simulink model "S_PARAM_V1"  (R2017a)
settings: Solver=VariableStepAuto  StartTime=0.0  StopTime=0.4  FixedStep=1e-6  MaxStep=1e-4  RelTol=1e-3
values from neighbouring files (symbols this model uses):
  a = 9    [M_PARAM_V1.m]    (also in M_PIL_PVSISTEM_2026_V1.m; ModTusk_V1.m)
  Alpha1 = 2*Zeta_obs*wn_obs    (= 2)    [M_PARAM_V1.m]    (also in M_PIL_PVSISTEM_2026_V1.m)
  Alpha2 = wn_obs    (= 1)    [M_PARAM_V1.m]    (also in M_PIL_PVSISTEM_2026_V1.m)
  alpha_max = 4/ts_min    (= 13333.3333333)    [M_PARAM_V1.m]    (also in M_PIL_PVSISTEM_2026_V1.m; ModTusk_V1.m)
  alpha_min = 4/ts_max    (= 259.067357513)    [M_PARAM_V1.m]    (also in M_PIL_PVSISTEM_2026_V1.m = 133.333333333; ModTusk_V1.m = 133.333333333)
  Cdc = Cdc    (= 0.0033)    [M_PARAM_V1.m]    (also in M_PIL_PVSISTEM_2026_V1.m = 0.00047)
  Cpv = Cpv    (= 0.0001)    [M_PARAM_V1.m]    (also in M_PIL_PVSISTEM_2026_V1.m = 0.0002)
  Epsilon = Ep_cont/Ts1    [M_PARAM_V1.m]    (also in M_PIL_PVSISTEM_2026_V1.m)
  ESRCdc = ESRCdc    (= 0.2)    [M_PARAM_V1.m]    (also in M_PIL_PVSISTEM_2026_V1.m)
  ESRCpv = ESRCpv    (= 0.2)    [M_PARAM_V1.m]    (also in M_PIL_PVSISTEM_2026_V1.m)
  K1 = Kt_acker_d    [M_PARAM_V1.m]    (also in M_PIL_PVSISTEM_2026_V1.m)
  K1y2md = Kmd(1:end-1)    [M_PARAM_V1.m]    (also in M_PIL_PVSISTEM_2026_V1.m)
  Kdpwm = 1/Ucmax    (= 0.000111111111111)    [M_PARAM_V1.m]    (also in M_PIL_PVSISTEM_2026_V1.m = 1.52590218967e-05)
  KI1 = Kp1/Ti1*Ts1    (= 760)    [M_PARAM_V1.m]    (also in M_PIL_PVSISTEM_2026_V1.m = 14.4)
  Kimd = -Kmd(end)    [M_PARAM_V1.m]    (also in M_PIL_PVSISTEM_2026_V1.m)
  KP1 = Kp1-KI1/2    (= 5320)    [M_PARAM_V1.m]    (also in M_PIL_PVSISTEM_2026_V1.m = 2392.8)
  L = L    (= 0.0044)    [M_PARAM_V1.m]    (also in M_PIL_PVSISTEM_2026_V1.m = 0.1)
  RL = RL    (= 0.494)    [M_PARAM_V1.m]    (also in M_PIL_PVSISTEM_2026_V1.m = 0.3)
  Ts = Ts1    (= 0.0002)    [M_PARAM_V1.m]    (also in M_PIL_PVSISTEM_2026_V1.m)
  Ts1 = 1/Fs    (= 0.0002)    [M_PARAM_V1.m]    (also in M_PIL_PVSISTEM_2026_V1.m)
  Ucmax = 9000    [M_PARAM_V1.m]    (also in M_PIL_PVSISTEM_2026_V1.m = 65535)
  vdc = 12    [M_PARAM_V1.m]    (also in M_PIL_PVSISTEM_2026_V1.m = 1000)
undefined symbols (not defined in the file or in its folder): Acid, Lead
undefined symbols (not defined in the file): Fs
libraries: powerlib x14, electricdrivelib x1, powerlib_meascontrol x1
settings Model: ExtModeTrigDuration=10  Creator=dricl  LastModifiedBy=dricl
settings OptimizationCC: PassReuseOutputArgsAs=Individual arguments  MaxStackSize=2560
settings DebuggingCC: ParameterTunabilityLossMsg=error
settings HardwareCC: ProdBitPerPointer=32  ProdBitPerSizeT=32  ProdBitPerPtrDiffT=32  ProdLargestAtomicInteger=Long  ProdLargestAtomicFloat=Double  ProdWordSize=32  ProdLongLongMode=on  ProdHWDeviceType=ARM Compatible->ARM Cortex
settings SFSimCC: MATLABDynamicMemAlloc=off
settings RTWCC: SystemTargetFile=ert.tlc  HardwareBoard=TI Concerto F28M35x (ARM Cortex-M3)  TLCOptions=-aInlineSetEventsForThisBaseRateFcn=TLC_FALSE -aSuppressMultiTaskScheduler=TLC_FALSE -aRateBasedStepFcn=1  TemplateMakefile=ert_default_tmf  Description=Embedded Coder  GenerateReport=on  Toolchain=Texas Instruments Code Composer Studio v6 (ARM)  IncludeHyperlinkInReport=on  LaunchReport=on  CreateSILPILBlock=PIL  GenerateTraceInfo=on  GenerateTraceReport=on  GenerateTraceReportSl=on  GenerateTraceReportSf=on  GenerateTraceReportEml=on
settings CodeAppCC: ForceParamTrailComments=on  IgnoreCustomStorageClasses=off  OperatorAnnotations=on  SimulinkDataObjDesc=on  SFDataObjDesc=on  MATLABFcnDesc=on  InsertBlockDesc=on  MATLABSourceComments=on

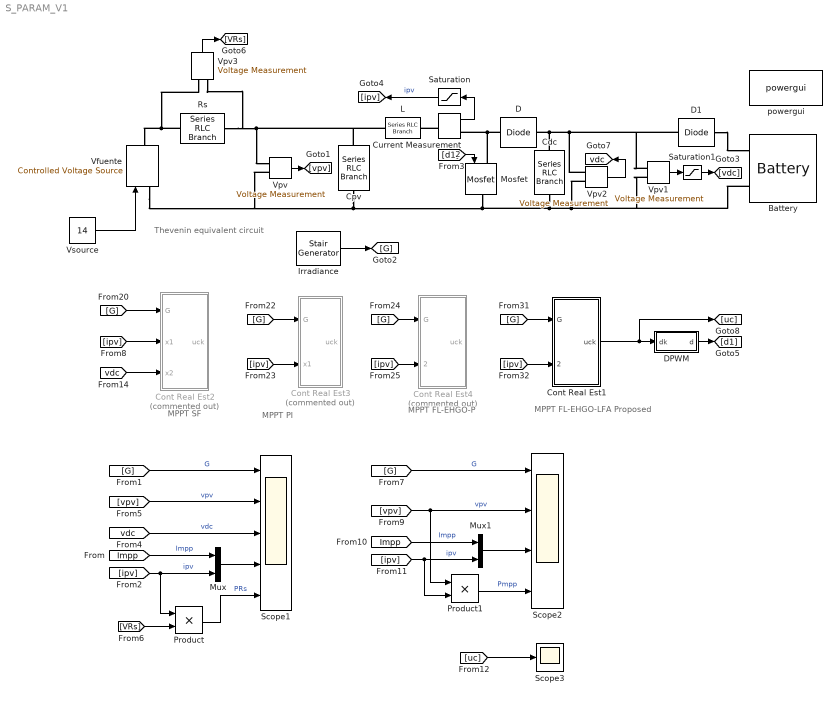
== system S_PARAM_V1 ==
  note: Thevenin equivalent circuit
  note: MPPT PI
  note: MPPT SF
  note: MPPT FL-EHGO-P
  note: MPPT FL-EHGO-LFA
      | Proposed
  Battery : electricdrivelib/Extra Sources/Battery  BatType=Lead-Acid  ShowTempParam=off  ThermalPreset=no  ShowAgeParam=off  NomV=12  NomQ=1.2  SOC=100  Batt_Tr=30  PresetModel=on  MaxQ=1.25  MinV=9  FullV=13.0658  Dis_rate=0.24  R=0.1  Normal_OP=0.37233  expZone="[12.2171        0.004]"  current=[6.5 13 32.5]  Units=Time  Tci=20  NomT=20  T2=-30  MaxQ2=4.8  FullV2=7.1  Normal_OP2=5.655  expZone2="[6.58           1]"  Rca=0.6  ti=2000  Dp=0  Neq0=0  Tsim=1e6  Ta1=25  Qeol=5.4*0.9  Reol=0.013333*1.2  Char_age=[2.3478, 3]  Dis_age=[2.3478, 10]  N1=1500  N2=10500  N3=1000  N4=1400  Ta2=45  N5=950
  Cdc : powerlib/Elements/Series RLC Branch  LConnTagsString=__new0  RConnTagsString=__new0  BranchType=RC  Resistance=ESRCdc  Inductance=1e-3  SetiL0=off  InitialCurrent=0  Capacitance=Cdc  Setx0=on  InitialVoltage=vdc_ref  Measurements=None
  Cont Real Est1 : Subsystem  Priority=7
  Cont Real Est2 : Subsystem  Priority=9  Commented=on
  Cont Real Est3 : Subsystem  Priority=7  Commented=on
  Cont Real Est4 : Subsystem  Priority=7  Commented=on
  Cpv : powerlib/Elements/Series RLC Branch  LConnTagsString=__new0  RConnTagsString=__new0  BranchType=RC  Resistance=ESRCpv  Inductance=1e-3  SetiL0=off  InitialCurrent=0  Capacitance=Cpv  Setx0=off  InitialVoltage=640.8  Measurements=None
  Current Measurement2 : powerlib/Measurements/Current Measurement  PhasorSimulation=off  OutputType=Complex  PSBequivalent=0
  D : powerlib/Power Electronics/Diode  Ron=Rondiode  Lon=0  Vf=Vfdiode  IC=0  UseSnubber=0  Rs=500  Cs=250e-9  Measurements=off
  D1 : powerlib/Power Electronics/Diode  Ron=0.001  Lon=0  Vf=0.7  IC=0  UseSnubber=0  Rs=500  Cs=250e-9  Measurements=off
  DPWM : Subsystem  AncestorBlock=plecslib_extras2/Modulators/Symmetrical PWM  mask(Symmetrical PWM){sampling=Natural (carrier starts with 0), fc=Fs, offset=0, input_limits=[0 Ucmax], output_values=[0 1]}
      mask prompts: fc "Carrier frequency (Hz):"; offset "Carrier offset (p.u.):"; input_limits "Input limits [min max]:"; output_values "Output values [off on]:"
      mask help: PWM generator with a symmetrical triangular carrier. If the input is a vector, the output is also a vector of the same width.
      mask init:
      | if numel(fc)>1 || fc<=0,
      |   error('Carrier frequency must be a positive scalar.');
      | end
      | if numel(offset)>1 || offset<0 || offset>=1,
      |   error('Carrier offset must be a scalar in the range [0; 1/fc[.');
      | end
      | if sampling == 1,
      |   offset = mod(offset+.75, 1);
      | end
      | 
      | si = [.5 mod(offset, .5)]/fc;
      mask Help: eval('plecs(''help'', ''symmetricalpwm.html'')')
      mask TypeOptions sampling: Natural (carrier starts with 0) | Natural (carrier starts with 1) | Regular (double edge) | Regular (single edge)
  Irradiance : powerlib_meascontrol/Pulse & Signal Generators/Stair Generator  t=[0, .1, .2, .3]  e=[0 1000 200 850]  Ts=0
      settings: SourceProductName=Simscape Power Systems
  L : powerlib/Elements/Series RLC Branch  LConnTagsString=__new0  RConnTagsString=__new0  BranchType=RL  Resistance=RL  Inductance=L  SetiL0=off  InitialCurrent=0  Capacitance=1e-6  Setx0=off  InitialVoltage=0  Measurements=None
  Mosfet : powerlib/Power Electronics/Mosfet  Ron=Ronfet  Lon=0  Rd=0  Vfd=0  IC=0  Rs=1e5  Cs=inf  Measurements=off
  Mux : Mux  Inputs=2
  Mux1 : Mux  Inputs=2
  Product : Product
  Product1 : Product
  Rs : powerlib/Elements/Series RLC Branch  LConnTagsString=__new0  RConnTagsString=__new0  BranchType=R  Resistance=2  Inductance=1e-3  SetiL0=off  InitialCurrent=0  Capacitance=Cpv  Setx0=off  InitialVoltage=640.8  Measurements=None
  Saturation : Saturate  UpperLimit=inf  LowerLimit=0
  Saturation1 : Saturate  UpperLimit=20  LowerLimit=0
  Scope1 : Scope  NumInputPorts=5
  Scope2 : Scope  NumInputPorts=4
  Scope3 : Scope
  Vfuente : powerlib/Electrical Sources/Controlled Voltage Source  Initialize=on  Source_Type=AC  Amplitude=0  Phase=0  Frequency=0  Measurements=None
  Vpv{,1..3} (4 alike) : powerlib/Measurements/Voltage Measurement  PhasorSimulation=off  OutputType=Complex  PSBequivalent=0
  Vsource : Constant  Value=14
  powergui : powerlib/powergui  Priority=1  SimulationMode=Continuous  SampleTime=50e-6  frequency=60  Iterations=50  frequencyindice=0  Pbase=100e6  ErrMax=1e-4  UnitsV=kV  UnitsW=MW  buscounter=0  FunctionMessages=off  echomessages=off  EnableUseOfTLC=off  CurrentSourceSwitches=off  DisableSnubberDevices=off  DisableRonSwitches=off  DisableVfSwitches=off  DisplayEquations=off  SolverType=Tustin/Backward Euler (TBE)  Interpol=off  ExternalGateDelay=off  methode=off  Ts=100  x0status=blocks  SPID=on  SwTol=0  HookPort=off  RestoreLinks=warning  ResistiveCurrentMeasurement=off  Frange=[0:2:500]  Ylog=off  Xlog=on  ShowGrid=off  save=off  variable=ZData  structure=0  ZoomFFT=off  StartTime=0.0  cycles=1  DisplayStyle=1  fundamental=60  FreqAxis=off  MaxFrequency=1000  frequencyindicesteady=1  RmsSteady=1  display=off
  tag scope: vdc=global
  wires:
  Vpv2/1 -> [vdc]
  DPWM/1(d) -> [d1]
  Saturation/1 -> [ipv]  "ipv"
  Vpv/1 -> [vpv]
  [d1] -> Mosfet/1
  Current Measurement2/1 -> Saturation/1
  [ipv] -> Product/1, Mux/2  "ipv"
  [Impp] -> Mux/1  "Impp"
  [G] -> Scope1/1  "G"
  Vpv1/1 -> Saturation1/1
  Saturation1/1 -> [vdc]
  [vdc] -> Scope1/3  "vdc"
  Mux/1 -> Scope1/4
  [vpv] -> Scope1/2  "vpv"
  Vpv3/1 -> [VRs]
  Product/1 -> Scope1/5  "PRs"
  [VRs] -> Product/2
  [Impp] -> Mux1/1  "Impp"
  [ipv] -> Product1/2, Mux1/2  "ipv"
  [G] -> Scope2/1  "G"
  [vpv] -> Product1/1, Scope2/2  "vpv"
  Mux1/1 -> Scope2/3
  Product1/1 -> Scope2/4  "Pmpp"
  Vsource/1 -> Vfuente/1
  Irradiance/1 -> [G]
  [G] -> Cont Real Est2/1(G)
  [ipv] -> Cont Real Est2/2(x1)
  [vdc] -> Cont Real Est2/3(x2)
  [ipv] -> Cont Real Est1/2(x1 = ipv)
  [G] -> Cont Real Est1/1(G)
  [uc] -> Scope3/1
  [G] -> Cont Real Est4/1(G)
  [ipv] -> Cont Real Est4/2(x1 = ipv)
  [G] -> Cont Real Est3/1(G)
  [ipv] -> Cont Real Est3/2(x1)
  Cont Real Est1/1(uck) -> [uc], DPWM/1(dk)
  connections:
  Cpv/LConn1 -- L/LConn1 -- Vpv3/LConn2 -- Rs/RConn1 -- Vpv/LConn1
  Cdc/RConn1 -- Vpv1/LConn2 -- Battery/LConn2 -- Vpv2/LConn2 -- Vfuente/LConn1 -- Vpv/LConn2 -- Cpv/RConn1 -- Mosfet/RConn1
  D/RConn1 -- Cdc/LConn1 -- Vpv1/LConn1 -- D1/LConn1 -- Vpv2/LConn1
  D/LConn1 -- Mosfet/LConn1 -- Current Measurement2/RConn1
  Current Measurement2/LConn1 -- L/RConn1
  D1/RConn1 -- Battery/LConn1
  Rs/LConn1 -- Vpv3/LConn1 -- Vfuente/RConn1

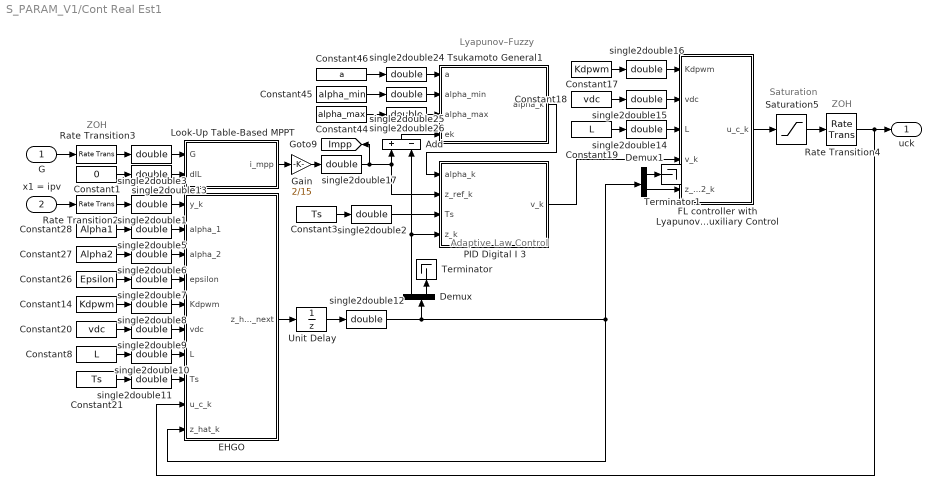
== system S_PARAM_V1/Cont Real Est1 ==
  note: Adaptive Law Control
  note: Lyapunov–Fuzzy
  note: ZOH
  note: Saturation
  note: ZOH
  G : Inport
  x1 = ipv : Inport  Port=2
  Add : Sum  Inputs=+-
  Constant1 : Constant  Value=0  SampleTime=Ts1
  Constant14 : Constant  Value=Kdpwm  SampleTime=Ts1
  Constant17 : Constant  Value=Kdpwm  SampleTime=Ts1
  Constant18 : Constant  Value=vdc  SampleTime=Ts1
  Constant19 : Constant  Value=L  SampleTime=Ts1
  Constant20 : Constant  Value=vdc  SampleTime=Ts1
  Constant21 : Constant  Value=Ts  SampleTime=Ts1
  Constant26 : Constant  Value=Epsilon  SampleTime=Ts1
  Constant27 : Constant  Value=Alpha2  SampleTime=Ts1
  Constant28 : Constant  Value=Alpha1  SampleTime=Ts1
  Constant3 : Constant  Value=Ts  SampleTime=Ts1
  Constant44 : Constant  Value=alpha_max  SampleTime=Ts1
  Constant45 : Constant  Value=alpha_min  SampleTime=Ts1
  Constant46 : Constant  Value=a  SampleTime=Ts1
  Constant8 : Constant  Value=L  SampleTime=Ts1
  Demux : Demux  Outputs=2
  Demux1 : Demux  Outputs=2
  EHGO : MATLAB Function  TreatAsAtomicUnit=on
  FL controller with Lyapunov–Fuzzy Adaptive Auxiliary Control : MATLAB Function  TreatAsAtomicUnit=on
  Gain : Gain  Gain=2/15
  Look-Up Table-Based MPPT : MATLAB Function  TreatAsAtomicUnit=on
  PID Digital I 3 : MATLAB Function  TreatAsAtomicUnit=on
  Rate Transition2 : RateTransition  Deterministic=off  OutPortSampleTime=Ts1
  Rate Transition3 : RateTransition  Deterministic=off  OutPortSampleTime=Ts1
  Rate Transition4 : RateTransition  Deterministic=off  OutPortSampleTime=Ts1
  Saturation5 : Saturate  UpperLimit=Ucmax  LowerLimit=0
  Terminator : Terminator
  Terminator1 : Terminator
  Tsukamoto General1 : MATLAB Function  TreatAsAtomicUnit=on
  Unit Delay : UnitDelay  SampleTime=Ts1
  single2double{1..3,5..17,24..26} (19 alike) : DataTypeConversion  OutDataTypeStr=double
  uck : Outport
  tag scope: Impp=global
  wires:
  FL controller with Lyapunov–Fuzzy Adaptive Auxiliary Control/1(u_c_k) -> Saturation5/1
  single2double1/1 -> EHGO/1(y_k)
  Rate Transition4/1 -> uck/1, EHGO/9(u_c_k)
  Constant28/1 -> single2double5/1
  single2double5/1 -> EHGO/2(alpha_1)
  Constant27/1 -> single2double6/1
  single2double6/1 -> EHGO/3(alpha_2)
  Constant26/1 -> single2double7/1
  single2double7/1 -> EHGO/4(epsilon)
  Constant14/1 -> single2double8/1
  single2double8/1 -> EHGO/5(Kdpwm)
  Constant20/1 -> single2double9/1
  single2double9/1 -> EHGO/6(vdc)
  Constant8/1 -> single2double10/1
  single2double10/1 -> EHGO/7(L)
  Constant21/1 -> single2double11/1
  single2double11/1 -> EHGO/8(Ts)
  Unit Delay/1 -> single2double12/1
  single2double12/1 -> Demux/1, Demux1/1, EHGO/10(z_hat_k)
  Constant19/1 -> single2double14/1
  Constant18/1 -> single2double15/1
  Constant17/1 -> single2double16/1
  single2double16/1 -> FL controller with Lyapunov–Fuzzy Adaptive Auxiliary Control/1(Kdpwm)
  single2double15/1 -> FL controller with Lyapunov–Fuzzy Adaptive Auxiliary Control/2(vdc)
  single2double14/1 -> FL controller with Lyapunov–Fuzzy Adaptive Auxiliary Control/3(L)
  EHGO/1(z_hat_next) -> Unit Delay/1
  Constant3/1 -> single2double2/1
  single2double2/1 -> PID Digital I 3/3(Ts)
  Constant46/1 -> single2double24/1
  single2double25/1 -> Tsukamoto General1/2(alpha_min)
  Constant44/1 -> single2double26/1
  single2double26/1 -> Tsukamoto General1/3(alpha_max)
  single2double24/1 -> Tsukamoto General1/1(a)
  Constant45/1 -> single2double25/1
  Add/1 -> Tsukamoto General1/4(ek)
  Demux/2 -> Terminator/1
  Demux/1 -> PID Digital I 3/4(z_k), Add/2
  Tsukamoto General1/1(alpha_k) -> PID Digital I 3/1(alpha_k)
  single2double3/1 -> Look-Up Table-Based MPPT/1(G)
  Constant1/1 -> single2double13/1
  single2double13/1 -> Look-Up Table-Based MPPT/2(dIL)
  Demux1/2 -> FL controller with Lyapunov–Fuzzy Adaptive Auxiliary Control/5(z_hat_2_k)
  Demux1/1 -> Terminator1/1
  PID Digital I 3/1(v_k) -> FL controller with Lyapunov–Fuzzy Adaptive Auxiliary Control/4(v_k)
  single2double17/1 -> [Impp], PID Digital I 3/2(z_ref_k), Add/1
  G/1 -> Rate Transition3/1
  x1 = ipv/1 -> Rate Transition2/1
  Rate Transition2/1 -> single2double1/1
  Rate Transition3/1 -> single2double3/1
  Saturation5/1 -> Rate Transition4/1
  Look-Up Table-Based MPPT/1(i_mpp) -> Gain/1
  Gain/1 -> single2double17/1

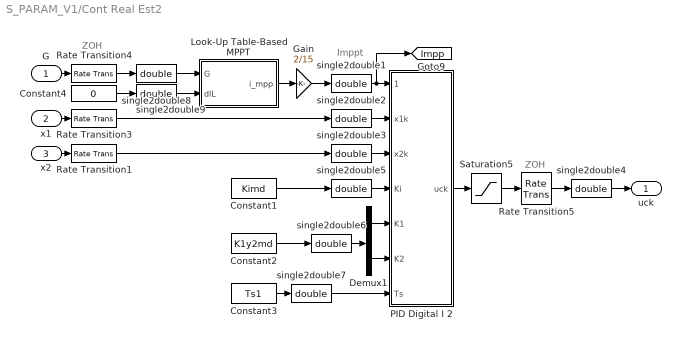
== system S_PARAM_V1/Cont Real Est2 ==
  note: Imppt
  note: ZOH
  note: ZOH
  G : Inport
  x1 : Inport  Port=2
  x2 : Inport  Port=3
  Constant1 : Constant  Value=Kimd  SampleTime=Ts1
  Constant2 : Constant  Value=K1y2md  SampleTime=Ts1
  Constant3 : Constant  Value=Ts1  SampleTime=Ts1
  Constant4 : Constant  Value=0  SampleTime=Ts1
  Demux1 : Demux  Outputs=2
  Gain : Gain  Gain=2/15
  Look-Up Table-Based MPPT : MATLAB Function  TreatAsAtomicUnit=on
  PID Digital I 2 : MATLAB Function  TreatAsAtomicUnit=on
  Rate Transition{1,3..5} (4 alike) : RateTransition  Deterministic=off  OutPortSampleTime=Ts1
  Saturation5 : Saturate  UpperLimit=Ucmax  LowerLimit=0
  single2double{1..9} (9 alike) : DataTypeConversion  OutDataTypeStr=double
  uck : Outport
  tag scope: Impp=global
  wires:
  PID Digital I 2/1(uck) -> Saturation5/1
  Constant1/1 -> single2double5/1
  Demux1/1 -> PID Digital I 2/5(K1)
  single2double1/1 -> [Impp], PID Digital I 2/1(x1k_Ref)
  single2double2/1 -> PID Digital I 2/2(x1k)
  single2double3/1 -> PID Digital I 2/3(x2k)
  single2double4/1 -> uck/1
  single2double5/1 -> PID Digital I 2/4(Ki)
  single2double7/1 -> PID Digital I 2/7(Ts)
  Constant4/1 -> single2double9/1
  single2double9/1 -> Look-Up Table-Based MPPT/2(dIL)
  single2double8/1 -> Look-Up Table-Based MPPT/1(G)
  single2double6/1 -> Demux1/1
  Demux1/2 -> PID Digital I 2/6(K2)
  Constant2/1 -> single2double6/1
  Constant3/1 -> single2double7/1
  Rate Transition4/1 -> single2double8/1
  G/1 -> Rate Transition4/1
  Rate Transition3/1 -> single2double2/1
  x1/1 -> Rate Transition3/1
  x2/1 -> Rate Transition1/1
  Rate Transition1/1 -> single2double3/1
  Saturation5/1 -> Rate Transition5/1
  Rate Transition5/1 -> single2double4/1
  Look-Up Table-Based MPPT/1(i_mpp) -> Gain/1
  Gain/1 -> single2double1/1

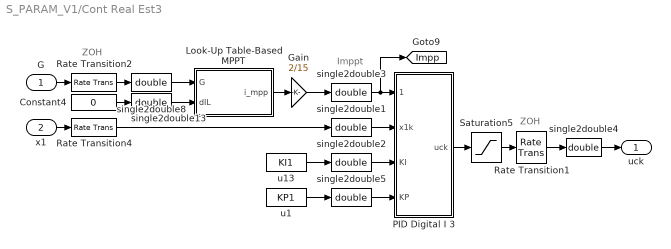
== system S_PARAM_V1/Cont Real Est3 ==
  note: Imppt
  note: ZOH
  note: ZOH
  G : Inport
  x1 : Inport  Port=2
  Constant4 : Constant  Value=0  SampleTime=Ts1
  Gain : Gain  Gain=2/15
  Look-Up Table-Based MPPT : MATLAB Function  TreatAsAtomicUnit=on
  PID Digital I 3 : MATLAB Function  TreatAsAtomicUnit=on
  Rate Transition1 : RateTransition  Deterministic=off  OutPortSampleTime=Ts1
  Rate Transition2 : RateTransition  Deterministic=off  OutPortSampleTime=Ts1
  Rate Transition4 : RateTransition  Deterministic=off  OutPortSampleTime=Ts1
  Saturation5 : Saturate  UpperLimit=Ucmax  LowerLimit=0
  single2double{1..5,8,13} (7 alike) : DataTypeConversion  OutDataTypeStr=double
  u1 : Constant  Value=KP1  SampleTime=Ts1
  u13 : Constant  Value=KI1  SampleTime=Ts1
  uck : Outport
  tag scope: Impp=global
  wires:
  u1/1 -> single2double5/1
  u13/1 -> single2double2/1
  PID Digital I 3/1(uck) -> Saturation5/1
  single2double3/1 -> [Impp], PID Digital I 3/1(x1k_ref)
  single2double1/1 -> PID Digital I 3/2(x1k)
  single2double4/1 -> uck/1
  single2double2/1 -> PID Digital I 3/3(KI)
  single2double5/1 -> PID Digital I 3/4(KP)
  single2double13/1 -> Look-Up Table-Based MPPT/2(dIL)
  Constant4/1 -> single2double13/1
  Look-Up Table-Based MPPT/1(i_mpp) -> Gain/1
  single2double8/1 -> Look-Up Table-Based MPPT/1(G)
  G/1 -> Rate Transition2/1
  Rate Transition2/1 -> single2double8/1
  x1/1 -> Rate Transition4/1
  Rate Transition4/1 -> single2double1/1
  Saturation5/1 -> Rate Transition1/1
  Rate Transition1/1 -> single2double4/1
  Gain/1 -> single2double3/1

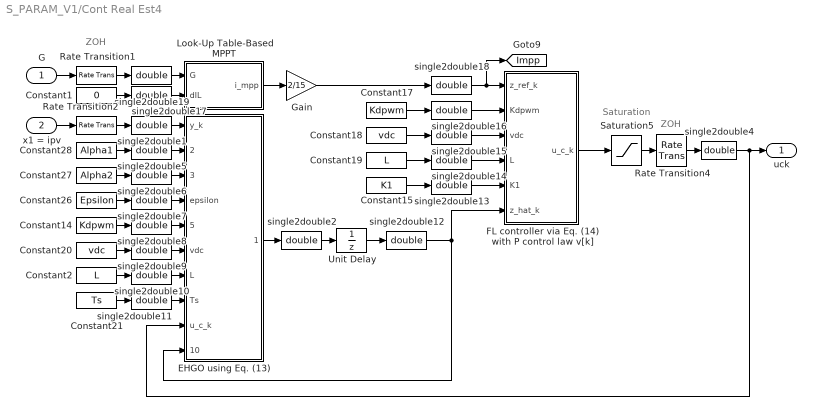
== system S_PARAM_V1/Cont Real Est4 ==
  note: Saturation
  note: ZOH
  note: ZOH
  G : Inport
  x1 = ipv : Inport  Port=2
  Constant1 : Constant  Value=0  SampleTime=Ts1
  Constant14 : Constant  Value=Kdpwm  SampleTime=Ts1
  Constant15 : Constant  Value=K1  SampleTime=Ts1
  Constant17 : Constant  Value=Kdpwm  SampleTime=Ts1
  Constant18 : Constant  Value=vdc  SampleTime=Ts1
  Constant19 : Constant  Value=L  SampleTime=Ts1
  Constant2 : Constant  Value=L  SampleTime=Ts1
  Constant20 : Constant  Value=vdc  SampleTime=Ts1
  Constant21 : Constant  Value=Ts  SampleTime=Ts1
  Constant26 : Constant  Value=Epsilon  SampleTime=Ts1
  Constant27 : Constant  Value=Alpha2  SampleTime=Ts1
  Constant28 : Constant  Value=Alpha1  SampleTime=Ts1
  EHGO using Eq. (13) : MATLAB Function  TreatAsAtomicUnit=on
  FL controller via Eq. (14) with P control law v[k] : MATLAB Function  TreatAsAtomicUnit=on
  Gain : Gain  Gain=2/15
  Look-Up Table-Based MPPT : MATLAB Function  TreatAsAtomicUnit=on
  Rate Transition1 : RateTransition  Deterministic=off  OutPortSampleTime=Ts1
  Rate Transition2 : RateTransition  Deterministic=off  OutPortSampleTime=Ts1
  Rate Transition4 : RateTransition  Deterministic=off  OutPortSampleTime=Ts1
  Saturation5 : Saturate  UpperLimit=Ucmax  LowerLimit=0
  Unit Delay : UnitDelay  SampleTime=Ts1
  single2double{1..2,4..19} (18 alike) : DataTypeConversion  OutDataTypeStr=double
  uck : Outport
  tag scope: Impp=global
  wires:
  FL controller via Eq. (14) with P control law v[k]/1(u_c_k) -> Saturation5/1
  single2double18/1 -> [Impp], FL controller via Eq. (14) with P control law v[k]/1(z_ref_k)
  single2double1/1 -> EHGO using Eq. (13)/1(y_k)
  single2double4/1 -> EHGO using Eq. (13)/9(u_c_k), uck/1
  Constant28/1 -> single2double5/1
  single2double5/1 -> EHGO using Eq. (13)/2(alpha_1)
  Constant27/1 -> single2double6/1
  single2double6/1 -> EHGO using Eq. (13)/3(alpha_2)
  Constant26/1 -> single2double7/1
  single2double7/1 -> EHGO using Eq. (13)/4(epsilon)
  Constant14/1 -> single2double8/1
  single2double8/1 -> EHGO using Eq. (13)/5(Kdpwm)
  Constant20/1 -> single2double9/1
  single2double9/1 -> EHGO using Eq. (13)/6(vdc)
  Constant2/1 -> single2double10/1
  single2double10/1 -> EHGO using Eq. (13)/7(L)
  Constant21/1 -> single2double11/1
  single2double11/1 -> EHGO using Eq. (13)/8(Ts)
  Unit Delay/1 -> single2double12/1
  single2double12/1 -> FL controller via Eq. (14) with P control law v[k]/6(z_hat_k), EHGO using Eq. (13)/10(z_hat_k)
  Constant15/1 -> single2double13/1
  Constant19/1 -> single2double14/1
  Constant18/1 -> single2double15/1
  Constant17/1 -> single2double16/1
  single2double16/1 -> FL controller via Eq. (14) with P control law v[k]/2(Kdpwm)
  single2double15/1 -> FL controller via Eq. (14) with P control law v[k]/3(vdc)
  single2double14/1 -> FL controller via Eq. (14) with P control law v[k]/4(L)
  single2double13/1 -> FL controller via Eq. (14) with P control law v[k]/5(K1)
  EHGO using Eq. (13)/1(z_hat_next) -> single2double2/1
  single2double2/1 -> Unit Delay/1
  Constant1/1 -> single2double17/1
  single2double17/1 -> Look-Up Table-Based MPPT/2(dIL)
  single2double19/1 -> Look-Up Table-Based MPPT/1(G)
  G/1 -> Rate Transition1/1
  x1 = ipv/1 -> Rate Transition2/1
  Rate Transition1/1 -> single2double19/1
  Rate Transition2/1 -> single2double1/1
  Saturation5/1 -> Rate Transition4/1
  Rate Transition4/1 -> single2double4/1
  Look-Up Table-Based MPPT/1(i_mpp) -> Gain/1
  Gain/1 -> single2double18/1

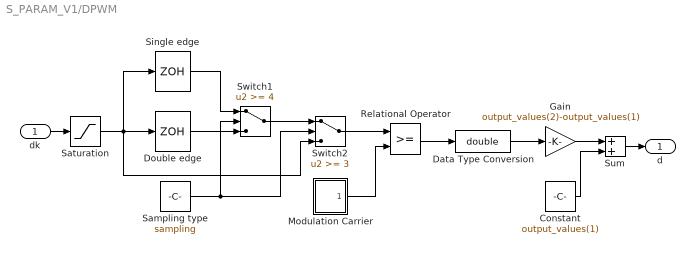
== system S_PARAM_V1/DPWM ==
  dk : Inport
  Constant : Constant  Value=output_values(1)
  Data Type Conversion : DataTypeConversion  OutDataTypeStr=double  SaturateOnIntegerOverflow=on  RndMeth=Zero
  Double edge : ZeroOrderHold  SampleTime=si
  Gain : Gain  Gain=output_values(2)-output_values(1)  SaturateOnIntegerOverflow=on  OutDataTypeStr=Inherit: Same as input  ParamDataTypeStr=Inherit: Same as input
  Modulation Carrier : Subsystem  mask(Symmetric Triangle Generator){fc=fc, offset=mod(offset+.5, 1), range=input_limits}
      mask prompts: fc "Carrier frequency (Hz):"; offset "Carrier offset (p.u.):"; range "Signal range [min max]:"
      mask help: Generates a symmetrical triangular signal with output values between 0 and 1. The block forces the Simulink solver to output all tips of the signal. The output can therefore be used as a carrier signal for PWM.
      mask init:
      | if numel(fc)>1 || fc<=0,
      |   error('Carrier frequency must be a positive scalar.');
      | end
      | if numel(offset)>1 || offset<0 || offset>=1,
      |   error('Carrier offset must be a scalar in the interval [0; 1[.');
      | end
      | if numel(range)~=2,
      |   error('Signal range must be a two-element vector.')
      | end
      | if range(1)>=range(2),
      |   error('Signal range must be specified as [min max].')
      | end
      | 
      | carrier_t = [0 offset mod(1/2+offset, 1) 1]/fc;
      | carrier_v0 = 1-2*abs(offset-.5);
      | carrier_v = range(1)+[carrier_v0 0 1 carrier_v0]*diff(range);
      | [carrier_t, idx] = unique(carrier_t);
      | carrier_v = carrier_v(idx);
      | si = [.5 mod(offset, .5)]/fc;
      | 
      | L = length(carrier_t);
      | disp_seq_t = repmat(carrier_t(:),1,3) + ones(L,1)*[0,1,2]/fc;
      | disp_seq_v = repmat(carrier_v(:),1,3);
      mask Display: plot(disp_seq_t, disp_seq_v)
  Relational Operator : RelationalOperator  RndMeth=Nearest  InputSameDT=on
  Sampling type : Constant  Value=sampling
  Saturation : Saturate  UpperLimit=input_limits(2)  LowerLimit=input_limits(1)
  Single edge : ZeroOrderHold  SampleTime=[1 offset]/fc
  Sum : Sum  SaturateOnIntegerOverflow=on  InputSameDT=on  OutDataTypeStr=Inherit: Same as first input
  Switch1 : Switch  Threshold=4  SaturateOnIntegerOverflow=on  InputSameDT=on
  Switch2 : Switch  Threshold=3  SaturateOnIntegerOverflow=on  InputSameDT=on
  d : Outport
  wires:
  Data Type Conversion/1 -> Gain/1
  Constant/1 -> Sum/2
  Gain/1 -> Sum/1
  Sum/1 -> d/1
  Relational Operator/1 -> Data Type Conversion/1
  Switch2/1 -> Relational Operator/1
  Sampling type/1 -> Switch1/2, Switch2/2
  Single edge/1 -> Switch1/1
  Saturation/1 -> Double edge/1, Single edge/1, Switch2/3
  dk/1 -> Saturation/1
  Modulation Carrier/1(Out) -> Relational Operator/2
  Switch1/1 -> Switch2/1
  Double edge/1 -> Switch1/3

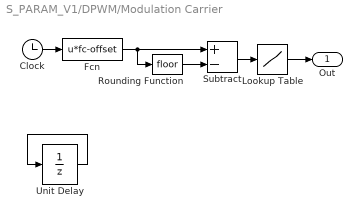
== system S_PARAM_V1/DPWM/Modulation Carrier ==
  Clock : Clock
  Fcn : Fcn  Expr=u*fc-offset
  Lookup Table : Lookup  InputValues=[0 .5 1]  Table=[range(1) range(2) range(1)]  LookUpMeth=Interpolation-Use End Values
  Rounding Function : Rounding
  Subtract : Sum  Inputs=+-
  Unit Delay : UnitDelay  SampleTime=si
  Out : Outport
  wires:
  Lookup Table/1 -> Out/1
  Subtract/1 -> Lookup Table/1
  Rounding Function/1 -> Subtract/2
  Fcn/1 -> Rounding Function/1, Subtract/1
  Clock/1 -> Fcn/1
  Unit Delay/1 -> Unit Delay/1

== matlab function S_PARAM_V1/Cont Real Est2/PID Digital I 2 ==
  data: x1k_Ref input; x1k input; x2k input; uck output; Ki input; K1 input; K2 input; Ts input
function uck = fcn(x1k_Ref, x1k, x2k, Ki, K1, K2, Ts)
% State-feedback controller with integral action used as a benchmark
% MPPT controller.
%
% Inputs:
%   x1k_Ref : current reference at sampling instant k
%   x1k     : first measured state at sampling instant k
%   x2k     : second measured state at sampling instant k
%   Ki      : integral gain
%   K1      : state-feedback gain associated with x1k
%   K2      : state-feedback gain associated with x2k
%   Ts      : sampling period
%
% Output:
%   uck     : control signal at sampling instant k

% Persistent variables used to preserve the controller states
% between consecutive sampling instants
persistent ek Acc_Int Acc_Int_1 uk

% Initialize persistent variables at the beginning of the simulation
if isempty(ek)
    ek = 0;
    Acc_Int = 0;
    Acc_Int_1 = 0;
    uk = 0;
end

% Tracking error
ek = x1k_Ref - x1k;

% Discrete-time integral action
Acc_Int = Ki * ek * Ts + Acc_Int_1;
Acc_Int_1 = Acc_Int;

% Control law: integral action combined with state feedback
uk = Acc_Int - (K1 * x1k + K2 * x2k);

% Controller output
uck = uk;

end

== matlab function S_PARAM_V1/Cont Real Est3/Look-Up Table-Based MPPT ==
  data: G input; i_mpp output; dIL input
function i_mpp = fcn(G, dIL)
% MPP current reference generation using a G-to-Impp lookup table.
%
% G       : irradiance input
% dIL     : peak-to-peak inductor-current ripple compensation
%
% Output:
% i_mpp   : compensated MPP current reference
%
% The lookup table covers G = 50...1200 W/m^2 with a 10 W/m^2 step.
% Linear interpolation is used within the table and extrapolation is
% applied outside the tabulated irradiance range.

persistent G_tab Impp_tab

if isempty(G_tab)

    G_tab = single(50:10:1200);

    Impp_tab = coder.const(double([ ...
    0.79 0.95 1.10 1.26 1.42 1.58 1.74 1.89 2.05 2.21 ...
    2.36 2.53 2.68 2.84 3.00 3.15 3.31 3.47 3.63 3.78 ...
    3.95 4.10 4.26 4.41 4.58 4.73 4.89 5.05 5.21 5.36 ...
    5.52 5.68 5.84 5.99 6.15 6.31 6.46 6.62 6.78 6.94 ...
    7.09 7.25 7.41 7.57 7.72 7.88 8.04 8.20 8.36 8.51 ...
    8.67 8.83 8.98 9.13 9.29 9.45 9.61 9.76 9.92 10.08 ...
    10.24 10.39 10.55 10.71 10.86 11.02 11.18 11.33 11.49 11.64 ...
    11.80 11.96 12.11 12.28 12.44 12.60 12.75 12.90 13.06 13.21 ...
    13.37 13.52 13.68 13.85 14.01 14.16 14.31 14.47 14.62 14.77 ...
    14.92 15.10 15.25 15.41 15.56 15.71 15.86 16.04 16.19 16.34 ...
    16.49 16.64 16.80 16.96 17.12 17.27 17.42 17.57 17.75 17.90 ...
    18.05 18.20 18.35 18.53 18.68 18.83
    ]));

end

% Nominal MPP-current interpolation
I_mpp_nom = interp1(G_tab, Impp_tab, G, 'linear', 'extrap');

% Inductor-current ripple compensation
i_mpp = I_mpp_nom - dIL;

% Prevent negative current-reference values
i_mpp = max(i_mpp, 0);

end

== matlab function S_PARAM_V1/Cont Real Est4/EHGO using Eq. (13) ==
  data: y_k input; alpha_1 input; alpha_2 input; epsilon input; Kdpwm input; vdc input; L input; Ts input; u_c_k input; z_hat_k input; z_hat_next output
function z_hat_next = fcn(y_k, alpha_1, alpha_2, epsilon, ...
                          Kdpwm, vdc, L, Ts, u_c_k, z_hat_k)
% Discrete-time extended high-gain observer (EHGO) used in the
% FL-EHGO structure with proportional auxiliary control.
%
% Inputs:
%   y_k        : measured output y[k] = i_pv[k]
%   alpha_1    : first EHGO coefficient
%   alpha_2    : second EHGO coefficient
%   epsilon    : EHGO tuning parameter
%   Kdpwm      : digital PWM gain
%   vdc        : dc-bus voltage
%   L          : boost-converter inductance
%   Ts         : sampling period
%   u_c_k      : converter control input u_c[k]
%   z_hat_k    : EHGO estimates [z_hat[k]; sigma_hat[k]]
%
% Output:
%   z_hat_next : EHGO estimates at k+1

z_hat_next = zeros(2,1);

% Observer estimation error
e_obs_k = y_k - z_hat_k(1);

% EHGO update according to Eq. (13)
% The nominal term b_hat is neglected in the practical implementation.

z_hat_next(1) = z_hat_k(1) + Ts * ( ...
    z_hat_k(2) + ...
    ((Kdpwm/L)*vdc)*u_c_k + ...
    (alpha_1/(epsilon*Ts))*e_obs_k );

z_hat_next(2) = z_hat_k(2) + Ts * ( ...
    (alpha_2/(epsilon^2*Ts^2))*e_obs_k );

end

== matlab function S_PARAM_V1/Cont Real Est4/FL controller via Eq. (14) with P control law v[k] ==
  data: z_ref_k input; Kdpwm input; vdc input; L input; K1 input; u_c_k output; z_hat_k input
function u_c_k = fcn(z_ref_k, Kdpwm, vdc, L, K1, z_hat_k)
% Feedback-linearizing control law with EHGO and proportional
% auxiliary control.
%
% This controller is used as the FL-EHGO benchmark for comparison
% with the proposed FL-EHGO structure with LFA control.
%
% Inputs:
%   z_ref_k   : tracking reference z_ref[k] = i_mpp[k]
%   Kdpwm     : digital PWM gain
%   vdc       : dc-bus voltage
%   L         : boost-converter inductance
%   K1        : proportional auxiliary-control gain
%   z_hat_k   : EHGO estimates [z_hat[k]; sigma_hat[k]]
%
% Output:
%   u_c_k     : converter control input u_c[k]

% EHGO estimates
z_est_k     = z_hat_k(1);
sigma_est_k = z_hat_k(2);

% Proportional auxiliary control
v_k = -K1 * (z_est_k - z_ref_k);

% Feedback-linearizing control input according to Eq. (14)
% The nominal term b_hat is neglected in the practical implementation.
u_c_k = (L/(Kdpwm*vdc)) * ...
        (-sigma_est_k + v_k);

end

== matlab function S_PARAM_V1/Cont Real Est4/Look-Up Table-Based MPPT ==
  data: G input; i_mpp output; dIL input
function i_mpp = fcn(G, dIL)
% MPP current reference generation using a G-to-Impp lookup table.
%
% G       : irradiance input
% dIL     : peak-to-peak inductor-current ripple compensation
%
% Output:
% i_mpp   : compensated MPP current reference
%
% The lookup table covers G = 50...1200 W/m^2 with a 10 W/m^2 step.
% Linear interpolation is used within the table and extrapolation is
% applied outside the tabulated irradiance range.

persistent G_tab Impp_tab

if isempty(G_tab)

    G_tab = single(50:10:1200);

    Impp_tab = coder.const(double([ ...
    0.79 0.95 1.10 1.26 1.42 1.58 1.74 1.89 2.05 2.21 ...
    2.36 2.53 2.68 2.84 3.00 3.15 3.31 3.47 3.63 3.78 ...
    3.95 4.10 4.26 4.41 4.58 4.73 4.89 5.05 5.21 5.36 ...
    5.52 5.68 5.84 5.99 6.15 6.31 6.46 6.62 6.78 6.94 ...
    7.09 7.25 7.41 7.57 7.72 7.88 8.04 8.20 8.36 8.51 ...
    8.67 8.83 8.98 9.13 9.29 9.45 9.61 9.76 9.92 10.08 ...
    10.24 10.39 10.55 10.71 10.86 11.02 11.18 11.33 11.49 11.64 ...
    11.80 11.96 12.11 12.28 12.44 12.60 12.75 12.90 13.06 13.21 ...
    13.37 13.52 13.68 13.85 14.01 14.16 14.31 14.47 14.62 14.77 ...
    14.92 15.10 15.25 15.41 15.56 15.71 15.86 16.04 16.19 16.34 ...
    16.49 16.64 16.80 16.96 17.12 17.27 17.42 17.57 17.75 17.90 ...
    18.05 18.20 18.35 18.53 18.68 18.83
    ]));

end

% Nominal MPP-current interpolation
I_mpp_nom = interp1(G_tab, Impp_tab, G, 'linear', 'extrap');

% Inductor-current ripple compensation
i_mpp = I_mpp_nom - dIL;

% Prevent negative current-reference values
i_mpp = max(i_mpp, 0);

end

== matlab function S_PARAM_V1/Cont Real Est3/PID Digital I 3 ==
  data: x1k_ref input; uck output; x1k input; KI input; KP input
function uck = fcn(x1k_ref, x1k, KI, KP)
% Discrete-time PI controller used as a benchmark MPPT controller.
%
% Inputs:
%   x1k_ref : current reference at sampling instant k
%   x1k     : measured current at sampling instant k
%   KI      : discrete integral gain
%   KP      : proportional gain
%
% Output:
%   uck     : control signal at sampling instant k

% Persistent variables used to store the current and previous
% error and control-signal values
persistent ek uk
persistent ek_1 uk_1

% Initialize persistent variables at the beginning of the simulation
if isempty(ek)
    ek = 0;
    uk = 0;
    ek_1 = 0;
    uk_1 = 0;
end

% Tracking error
ek = x1k_ref - x1k;

% Incremental discrete-time PI control law
uk = ek*(KP + KI) - ek_1*KP + uk_1;

% Store current values for the next sampling instant
ek_1 = ek;
uk_1 = uk;

% Controller output
uck = uk;

end

== matlab function S_PARAM_V1/Cont Real Est2/Look-Up Table-Based MPPT ==
  data: G input; i_mpp output; dIL input
function i_mpp = fcn(G, dIL)
% MPP current reference generation using a G-to-Impp lookup table.
%
% G       : irradiance input
% dIL     : peak-to-peak inductor-current ripple compensation
%
% Output:
% i_mpp   : compensated MPP current reference
%
% The lookup table covers G = 50...1200 W/m^2 with a 10 W/m^2 step.
% Linear interpolation is used within the table and extrapolation is
% applied outside the tabulated irradiance range.

persistent G_tab Impp_tab

if isempty(G_tab)

    G_tab = single(50:10:1200);

    Impp_tab = coder.const(double([ ...
    0.79 0.95 1.10 1.26 1.42 1.58 1.74 1.89 2.05 2.21 ...
    2.36 2.53 2.68 2.84 3.00 3.15 3.31 3.47 3.63 3.78 ...
    3.95 4.10 4.26 4.41 4.58 4.73 4.89 5.05 5.21 5.36 ...
    5.52 5.68 5.84 5.99 6.15 6.31 6.46 6.62 6.78 6.94 ...
    7.09 7.25 7.41 7.57 7.72 7.88 8.04 8.20 8.36 8.51 ...
    8.67 8.83 8.98 9.13 9.29 9.45 9.61 9.76 9.92 10.08 ...
    10.24 10.39 10.55 10.71 10.86 11.02 11.18 11.33 11.49 11.64 ...
    11.80 11.96 12.11 12.28 12.44 12.60 12.75 12.90 13.06 13.21 ...
    13.37 13.52 13.68 13.85 14.01 14.16 14.31 14.47 14.62 14.77 ...
    14.92 15.10 15.25 15.41 15.56 15.71 15.86 16.04 16.19 16.34 ...
    16.49 16.64 16.80 16.96 17.12 17.27 17.42 17.57 17.75 17.90 ...
    18.05 18.20 18.35 18.53 18.68 18.83
    ]));

end

% Nominal MPP-current interpolation
I_mpp_nom = interp1(G_tab, Impp_tab, G, 'linear', 'extrap');

% Inductor-current ripple compensation
i_mpp = I_mpp_nom - dIL;

% Prevent negative current-reference values
i_mpp = max(i_mpp, 0);

end

== matlab function S_PARAM_V1/Cont Real Est1/EHGO ==
  data: y_k input; alpha_1 input; alpha_2 input; epsilon input; Kdpwm input; vdc input; L input; Ts input; u_c_k input; z_hat_k input; z_hat_next output
function z_hat_next = fcn(y_k, alpha_1, alpha_2, epsilon, ...
                          Kdpwm, vdc, L, Ts, u_c_k, z_hat_k)
% Discrete-time extended high-gain observer (EHGO).
%
% Inputs:
%   y_k       : measured output y[k]
%   alpha_1   : first EHGO coefficient
%   alpha_2   : second EHGO coefficient
%   epsilon   : high-gain observer tuning parameter
%   Kdpwm     : DPWM gain
%   vdc       : dc-bus voltage
%   L         : Boost-converter inductance
%   Ts        : sampling period
%   u_c_k     : converter control input u_c[k]
%   z_hat_k   : current EHGO state estimates
%
% Output:
%   z_hat_next : EHGO state estimates at k+1

z_hat_next = zeros(2,1);

% Output-estimation error
e_obs_k = y_k - z_hat_k(1);

% EHGO state update
z_hat_next(1) = z_hat_k(1) + Ts * ( ...
    z_hat_k(2) + ...
    ((Kdpwm/L)*vdc)*u_c_k + ...
    (alpha_1/(epsilon*Ts))*e_obs_k );

z_hat_next(2) = z_hat_k(2) + Ts * ( ...
    (alpha_2/(epsilon^2*Ts^2))*e_obs_k );

end

== matlab function S_PARAM_V1/Cont Real Est1/FL controller with Lyapunov–Fuzzy Adaptive Auxiliary Control ==
  data: Kdpwm input; vdc input; L input; v_k input; u_c_k output; z_hat_2_k input
function u_c_k = fcn(Kdpwm, vdc, L, v_k, z_hat_2_k)
% Feedback-linearizing control law using the EHGO estimate.
%
% Inputs:
%   Kdpwm       : DPWM gain
%   vdc         : dc-bus voltage
%   L           : Boost-converter inductance
%   v_k         : LFA auxiliary control v[k]
%   z_hat_2_k   : second EHGO state estimate
%
% Output:
%   u_c_k       : converter control input u_c[k]

u_c_k = (L/(Kdpwm*vdc)) * ...
        (-z_hat_2_k + v_k);

end

== matlab function S_PARAM_V1/Cont Real Est1/Look-Up Table-Based MPPT ==
  data: G input; i_mpp output; dIL input
function i_mpp = fcn(G, dIL)
% MPP current reference generation using a G-to-Impp lookup table.
%
% G       : irradiance input
% dIL     : peak-to-peak inductor-current ripple compensation
%
% Output:
% i_mpp   : compensated MPP current reference
%
% The lookup table covers G = 50...1200 W/m^2 with a 10 W/m^2 step.
% Linear interpolation is used within the table and extrapolation is
% applied outside the tabulated irradiance range.

persistent G_tab Impp_tab

if isempty(G_tab)

    G_tab = single(50:10:1200);

    Impp_tab = coder.const(double([ ...
    0.79 0.95 1.10 1.26 1.42 1.58 1.74 1.89 2.05 2.21 ...
    2.36 2.53 2.68 2.84 3.00 3.15 3.31 3.47 3.63 3.78 ...
    3.95 4.10 4.26 4.41 4.58 4.73 4.89 5.05 5.21 5.36 ...
    5.52 5.68 5.84 5.99 6.15 6.31 6.46 6.62 6.78 6.94 ...
    7.09 7.25 7.41 7.57 7.72 7.88 8.04 8.20 8.36 8.51 ...
    8.67 8.83 8.98 9.13 9.29 9.45 9.61 9.76 9.92 10.08 ...
    10.24 10.39 10.55 10.71 10.86 11.02 11.18 11.33 11.49 11.64 ...
    11.80 11.96 12.11 12.28 12.44 12.60 12.75 12.90 13.06 13.21 ...
    13.37 13.52 13.68 13.85 14.01 14.16 14.31 14.47 14.62 14.77 ...
    14.92 15.10 15.25 15.41 15.56 15.71 15.86 16.04 16.19 16.34 ...
    16.49 16.64 16.80 16.96 17.12 17.27 17.42 17.57 17.75 17.90 ...
    18.05 18.20 18.35 18.53 18.68 18.83
    ]));

end

% Nominal MPP-current interpolation
I_mpp_nom = interp1(G_tab, Impp_tab, G, 'linear', 'extrap');

% Inductor-current ripple compensation
i_mpp = I_mpp_nom - dIL;

% Prevent negative current-reference values
i_mpp = max(i_mpp, 0);

end

== matlab function S_PARAM_V1/Cont Real Est1/PID Digital I 3 ==
  data: alpha_k input; z_ref_k input; Ts input; v_k output; z_k input
function v_k = fcn(alpha_k, z_ref_k, Ts, z_k)
% LFA auxiliary control implementation.
%
% The decay rate alpha[k], provided by the two-rule Tsukamoto fuzzy
% inference system, determines the discrete-time contraction factor
% lambda[k]. The adaptive gains K[k] and L[k] are then computed to
% generate the auxiliary control v[k].
%
% Inputs:
%   alpha_k : Decay rate alpha[k] provided by the fuzzy inference system
%   z_ref_k : Tracking reference z_ref[k] = i_mpp[k]
%   Ts      : Sampling period
%   z_k     : Feedback-linearized state z[k]
%
% Output:
%   v_k     : Auxiliary control v[k]

% Numerical protection
alpha_k = max(alpha_k, eps);

% Contraction factor - equation (35)
lambda_k = exp(-alpha_k * Ts);

% Adaptive auxiliary-control gains - equation (34)
K_k = (1 - lambda_k) / Ts;
L_k = (1 - lambda_k) / Ts;

% LFA auxiliary control law - equation (34)
v_k = -K_k * z_k + L_k * z_ref_k;

end

== matlab function S_PARAM_V1/Cont Real Est1/Tsukamoto General1 ==
  data: a input; alpha_min input; alpha_max input; ek input; alpha_k output
function alpha_k = fcn(a, alpha_min, alpha_max, ek)
% General two-rule Tsukamoto implementation with w1 = exp(...)
%
% ek         : tracking error (scalar or vector)
% a          : Gaussian width parameter for mu_A1(|ek|)
% alpha_min  : lower bound of the physical decay-rate interval
% alpha_max  : upper bound of the physical decay-rate interval
%
% Output:
% alpha_k    : decay rate alpha[k] in [alpha_min, alpha_max]

% Numerical protection
a = max(a, eps);

% Width of the physical decay-rate interval
Delta_alpha = alpha_max - alpha_min;

% Centered output universe
alpha_c_min = -Delta_alpha/2;
alpha_c_max =  Delta_alpha/2;

% Input fuzzification based on the tracking-error magnitude
e_abs = abs(ek);

w1 = exp(-(e_abs.^2)/(2*a^2));   % mu_A1(|ek|): small tracking error
w2 = 1 - w1;                     % mu_A2(|ek|): large tracking error

% Tsukamoto inversion for alpha_c in
% [alpha_c_min, alpha_c_max]
z1 = alpha_c_max - w1.*Delta_alpha;  % R1: A1 -> B2 (decreasing)
z2 = alpha_c_min + w2.*Delta_alpha;  % R2: A2 -> B1 (increasing)

% Normalized weighted aggregation in the centered universe
den = w1 + w2;
den(den < eps) = eps;

alpha_c = ...
    (w1.*z1 + w2.*z2) ./ den;

% Translation to the physical decay-rate interval
alpha_k = ...
    alpha_c + ...
    (alpha_min + alpha_max)/2;

% Optional numerical saturation
alpha_k = ...
    min(max(alpha_k, alpha_min), alpha_max);

end
